simulink model "dc_motor_sys_id_MIO_16E4_2015a"  (R2015a)
settings: Solver=ode3  SolverMode=SingleTasking  StartTime=0.0  StopTime=5  RelTol=1e-3
model workspace (MAT data in the model file):
  freq = 0
values from neighbouring files (symbols this model uses):
  a = 37.04    [ControlSystemDesigner_e_Nyquist.m]    (also in ex3_5.m)
  k0 = 1.382    [ControlSystemDesigner_e_Nyquist.m]
undefined symbols (not defined in the file or in its folder): MIO, National_Instruments, PCI
libraries: sldrtlib x5
settings Model: SimulationMode=external  ExtModeTrigDuration=60001  Creator=Alunos  LastModifiedBy=alunos
settings OptimizationCC: BlockReduction=off  BooleanDataType=off
settings DebuggingCC: SaveWithParameterizedLinksMsg=none  UnderspecifiedInitializationDetection=Classic  MergeDetectMultiDrivingBlocksExec=none  SignalResolutionControl=TryResolveAllWithWarning
settings HardwareCC: ProdIntDivRoundTo=Zero  ProdEndianess=LittleEndian  ProdHWDeviceType=Intel->x86/Pentium  TargetIntDivRoundTo=Zero  TargetEndianess=LittleEndian  TargetHWDeviceType=Intel->x86/Pentium
settings RTWCC: SystemTargetFile=rtwin.tlc  TemplateMakefile=rtwin.tmf  Description=Simulink Desktop Real-Time  RTWCompilerOptimization=on
settings CodeAppCC: MaxIdLength=95
settings TargetCC: TargetPreCompLibLocation=C:\Program Files\MATLAB\R2015a\toolbox\sldrt\lib\win32

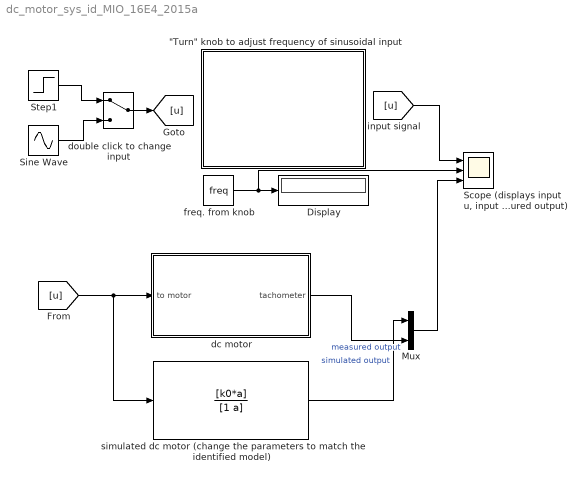
== system dc_motor_sys_id_MIO_16E4_2015a ==
  "\"Turn\" knob to adjust frequency of sinusoidal input" : Subsystem  DialogController=hmiCreateDDGDialog  IsWebBlock=on  mask(MathWorksWebBlock){webBlockId=642ff565-5490-4939-a910-963d1c1b9544, webBlockType=continuousknob, ShowInLibBrowser=on, ShowInitialText=on, HMISrcModelName=dc_motor_modeling_MIO_16E4_2015a}
      mask prompts: webBlockId "WebBlock Id"; webBlockType "WebBlock Type"; HMISrcModelName "Source Model"
      mask help: Set a value to tune parameters or variables.
      mask Help: helpview([docroot '/mapfiles/simulink.map'], 'hmi_knob')
      mask Display:
      | if strcmp(get_param(bdroot(gcb),'BlockDiagramType'),'library')
      |  image([(matlabroot) '/toolbox/simulink/hmi/icons/ContinuousKnob.png'])
      | end
  Display : Display
  Mux : Mux  Inputs=2
  "Scope (displays input u, input frequency, simulated output, and measured output)" : Scope  NumInputPorts=3
      settings: ShowLegends=on  TimeRange=5  YMin=0~-1~-0.5  YMax=1~1~1.5
  Sine Wave : Sin  Amplitude=0.5  Frequency=freq  SampleTime=0
  Step1 : Step  SampleTime=0
  dc motor : Subsystem
  double click to change input : ManualSwitch
  "freq. from knob " : Constant  Value=freq
  simulated dc motor (change the parameters to match the identified model) : TransferFcn  Numerator=[k0*a]  Denominator=[1 a]
  wires:
  Step1/1 -> double click to change input/1
  Sine Wave/1 -> double click to change input/2
  double click to change input/1 -> [u]
  [u] -> dc motor/1(to motor), simulated dc motor (change the parameters to match the identified model)/1
  [u] -> "Scope (displays input u, input frequency, simulated output, and measured output)"/1
  simulated dc motor (change the parameters to match the identified model)/1 -> Mux/1  "simulated output"
  dc motor/1(tachometer) -> Mux/2  "measured output"
  Mux/1 -> "Scope (displays input u, input frequency, simulated output, and measured output)"/3
  "freq. from knob "/1 -> "Scope (displays input u, input frequency, simulated output, and measured output)"/2, Display/1

== system dc_motor_sys_id_MIO_16E4_2015a/"Turn" knob to adjust frequency of sinusoidal input ==

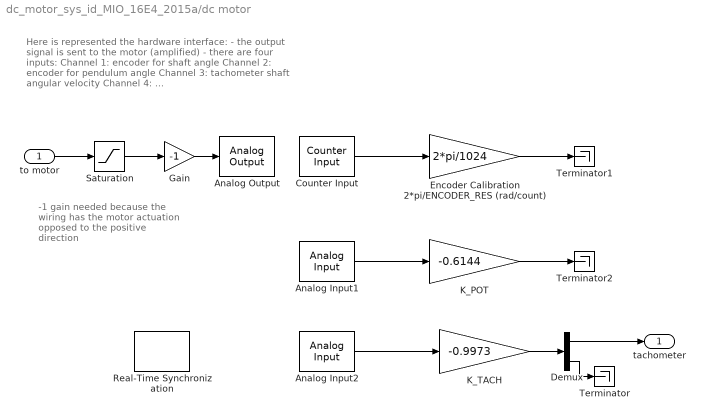
== system dc_motor_sys_id_MIO_16E4_2015a/dc motor ==
  note: -1 gain needed
      | because the wiring
      | has the motor
      | actuation opposed to
      | the positive direction
  note: Here is represented the hardware interface:
      | - the output signal is sent to the motor (amplified)
      | - there are four inputs:
      | Channel 1: encoder for shaft angle
      | Channel 2: encoder for pendulum angle
      | Channel 3: tachometer shaft angular velocity
      | Channel 4: ...
  to motor : Inport
  Analog Input1 : sldrtlib/Analog Input  SampleTime=0.001  MaxMissedTicks=10  ShowMissedTicks=off  YieldWhenWaiting=off  DrvName=National_Instruments/PCI-MIO-16E-4  DrvAddress=4294967295  DrvOptions=[0 0 0 0 1 0]  Channels=1:2  RangeMode=1  VoltRange=1  DataType=1
      settings: AttributesFormatString=National Instruments\nPCI-MIO-16E-4 [auto]
  Analog Input2 : sldrtlib/Analog Input  SampleTime=0.001  MaxMissedTicks=10  ShowMissedTicks=off  YieldWhenWaiting=off  DrvName=National_Instruments/PCI-MIO-16E-4  DrvAddress=4294967295  DrvOptions=[0 0 0 0 1 0]  Channels=3:4  RangeMode=1  VoltRange=1  DataType=1
      settings: AttributesFormatString=National Instruments\nPCI-MIO-16E-4 [auto]
  Analog Output : sldrtlib/Analog Output  SampleTime=0.001  MaxMissedTicks=inf  ShowMissedTicks=off  YieldWhenWaiting=off  DrvName=National_Instruments/PCI-MIO-16E-4  DrvAddress=4294967295  DrvOptions=[0 0 0 0 1 0]  Channels=1  RangeMode=1  VoltRange=1  InitialValue=[]  FinalValue=0
      settings: AttributesFormatString=National Instruments\nPCI-MIO-16E-4 [auto]
  Counter Input : sldrtlib/Counter Input  SampleTime=0.001  MaxMissedTicks=inf  ShowMissedTicks=off  YieldWhenWaiting=off  DrvName=National_Instruments/PCI-MIO-16E-4  DrvAddress=4294967295  DrvOptions=[0 0 0 0 1 0]  Channels=1:2  ResetMode=1  CounterEdge=1  CounterGate=1  DataType=1
      settings: AttributesFormatString=National Instruments\nPCI-MIO-16E-4 [auto]
  Demux : Demux  Outputs=2
  Encoder Calibration 2*pi/ENCODER_RES (rad/count) : Gain  Gain=2*pi/1024  SaturateOnIntegerOverflow=on  OutDataTypeStr=Inherit: Same as input  ParamDataTypeStr=Inherit: Same as input
  Gain : Gain  Gain=-1
  K_POT : Gain  Gain=-0.6144  SaturateOnIntegerOverflow=on  OutDataTypeStr=Inherit: Same as input  ParamDataTypeStr=Inherit: Same as input
  "K_TACH " : Gain  Gain=-0.9973  SaturateOnIntegerOverflow=on  OutDataTypeStr=Inherit: Same as input  ParamDataTypeStr=Inherit: Same as input
  Real-Time Synchronization : sldrtlib/Real-Time Synchronization  SampleTime=0.001  MaxMissedTicks=inf  ShowMissedTicks=off  YieldWhenWaiting=off
  Saturation : Saturate  UpperLimit=10  LowerLimit=-10
  Terminator : Terminator
  Terminator1 : Terminator
  Terminator2 : Terminator
  tachometer : Outport
  wires:
  Analog Input1/1 -> K_POT/1
  Gain/1 -> Analog Output/1
  Counter Input/1 -> Encoder Calibration 2*pi/ENCODER_RES (rad/count)/1
  Analog Input2/1 -> "K_TACH "/1
  "K_TACH "/1 -> Demux/1
  Demux/1 -> tachometer/1
  Demux/2 -> Terminator/1
  to motor/1 -> Saturation/1
  Saturation/1 -> Gain/1
  Encoder Calibration 2*pi/ENCODER_RES (rad/count)/1 -> Terminator1/1
  K_POT/1 -> Terminator2/1
